simulink model "lab3_integration"  (R2020a)
settings: Solver=VariableStepAuto  StartTime=0.0  StopTime=10.0  RelTol=1e-3
libraries: androidsensorlib x3, sharedTrackingLibrary x1
settings Model: Creator=horia  LastModifiedBy=horia

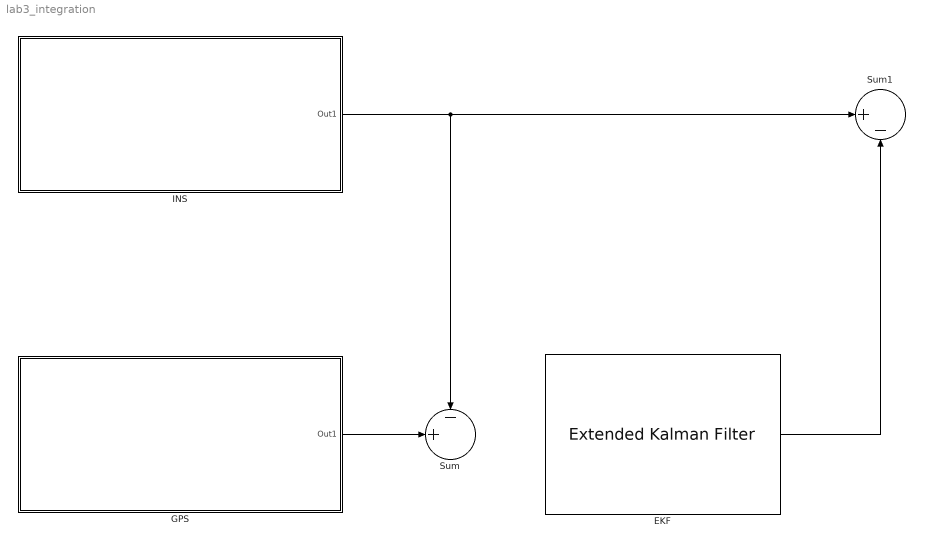
== system lab3_integration ==
  EKF : sharedTrackingLibrary/Extended Kalman Filter  StateTransitionFcn=myStateTransitionFcn  HasStateTransitionJacobianFcn=off  HasAdditiveProcessNoise=Additive  ProcessNoise=1  HasTimeVaryingProcessNoise=off  HasStateTransitionFcnExtraArgument=0  InitialState=0  InitialStateCovariance=1  MeasurementFcn1=myMeasurementFcn  HasMeasurementJacobianFcn1=off  HasMeasurementEnablePort1=off  HasAdditiveMeasurementNoise1=Additive  MeasurementNoise1=1  HasTimeVaryingMeasurementNoise1=off  HasMeasurementFcnExtraArgument1=0  MeasurementFcn2=myMeasurementFcn  HasMeasurementJacobianFcn2=off  HasMeasurementEnablePort2=off  HasAdditiveMeasurementNoise2=Additive  MeasurementNoise2=1  HasTimeVaryingMeasurementNoise2=off  HasMeasurementFcnExtraArgument2=0  MeasurementFcn3=myMeasurementFcn  HasMeasurementJacobianFcn3=off  HasMeasurementEnablePort3=off  HasAdditiveMeasurementNoise3=Additive  MeasurementNoise3=1  HasTimeVaryingMeasurementNoise3=off  HasMeasurementFcnExtraArgument3=0  MeasurementFcn4=myMeasurementFcn  HasMeasurementJacobianFcn4=off  HasMeasurementEnablePort4=off  HasAdditiveMeasurementNoise4=Additive  MeasurementNoise4=1  HasTimeVaryingMeasurementNoise4=off  HasMeasurementFcnExtraArgument4=0  MeasurementFcn5=myMeasurementFcn  HasMeasurementJacobianFcn5=off  HasMeasurementEnablePort5=off  HasAdditiveMeasurementNoise5=Additive  MeasurementNoise5=1  HasTimeVaryingMeasurementNoise5=off  HasMeasurementFcnExtraArgument5=0  EnableMultirate=off  StateTransitionFcnSampleTime=1  MeasurementFcn1SampleTime=1  MeasurementFcn2SampleTime=1  MeasurementFcn3SampleTime=1  MeasurementFcn4SampleTime=1  MeasurementFcn5SampleTime=1  UseCurrentEstimator=on  OutputStateCovariance=off  DataType=double  SampleTime=1  NumberOfMeasurements=2
      settings: SourceProductBaseCode=CT,DR,TF,ID,NV,AR,RO,VE
  GPS : Subsystem
  INS : Subsystem
  Sum : Sum  Inputs=-+|
  Sum1 : Sum  Inputs=|+-
  wires:
  GPS/1(Out1) -> Sum/2
  INS/1(Out1) -> Sum1/1, Sum/1
  EKF/1 -> Sum1/2

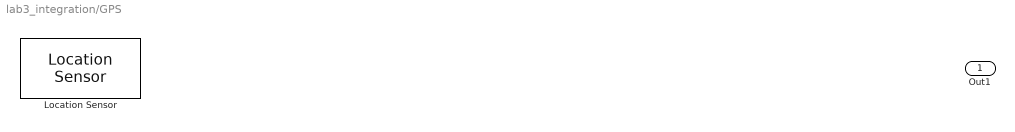
== system lab3_integration/GPS ==
  Location Sensor : androidsensorlib/Location Sensor  OutputVector=off  SampleTime=0.1  BlockPlatform=Android
      settings: SourceProductBaseCode=ANDROID
  Out1 : Outport

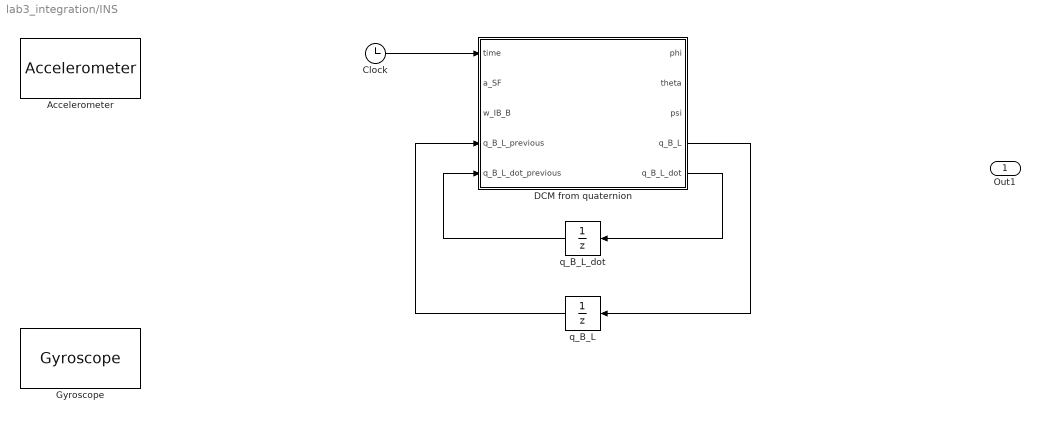
== system lab3_integration/INS ==
  Accelerometer : androidsensorlib/Accelerometer  OutputVector=off  SampleTime=0.1  BlockPlatform=Android
      settings: SourceProductBaseCode=ANDROID
  Clock : Clock
  DCM from quaternion : MATLAB Function  TreatAsAtomicUnit=on
  Gyroscope : androidsensorlib/Gyroscope  OutputVector=off  SampleTime=0.1  BlockPlatform=Android
      settings: SourceProductBaseCode=ANDROID
  q_B_L : UnitDelay  InitialCondition=[1;0;0;0]  SampleTime=-1  HasFrameUpgradeWarning=on
  q_B_L_dot : UnitDelay  InitialCondition=zeros(4,1)  SampleTime=-1  HasFrameUpgradeWarning=on
  Out1 : Outport
  wires:
  q_B_L_dot/1 -> DCM from quaternion/5(q_B_L_dot_previous)
  DCM from quaternion/4(q_B_L) -> q_B_L/1
  DCM from quaternion/5(q_B_L_dot) -> q_B_L_dot/1
  q_B_L/1 -> DCM from quaternion/4(q_B_L_previous)
  Clock/1 -> DCM from quaternion/1(time)

== matlab function lab3_integration/INS/DCM from quaternion ==
  data: time input; a_SF input; phi output; w_IB_B input; theta output; psi output; q_B_L_previous input; q_B_L_dot_previous input; q_B_L output; q_B_L_dot output
function [phi,theta,psi,q_B_L,q_B_L_dot] = fcn(time,a_SF,w_IB_B,q_B_L_previous,q_B_L_dot_previous)
%-- Partie initialisation ---------------------
persistent FlagInit counteur
theta = 0;
phi = 0;
psi = 0;
q_B_L = q_B_L_previous ;
q_B_L_dot = q_B_L_dot_previous  ;
a_SF_sum = zeros(1,3);

%%%%%%%%%%%%%%%%%%%%%%%%%%%%%%%%%%%%%%%%%%%%%%%%%%%%%%%%%%%%%%%%%%%%%%%%%%%
%
%  function R=q2dcm(q)
%
%>
%> @brief Function that converts a  quaternion vector to a directional
%> cosine matrix (rotation matrix) 
%>
%> @param[out]   R      Rotation matrix.
%> @param[in]    q      Quaternion vector.
%>
%
%%%%%%%%%%%%%%%%%%%%%%%%%%%%%%%%%%%%%%%%%%%%%%%%%%%%%%%%%%%%%%%%%%%%%%%%%%%
function R=q2dcm(q)

R = zeros(3,3);
p=zeros(6,1);

p(1:4)=q.^2;

p(5)=p(2)+p(3);

if p(1)+p(4)+p(5)~=0
   p(6)=2/(p(1)+p(4)+p(5)); 
else
   p(6)=0;
end


R(1,1)=1-p(6)*p(5);
R(2,2)=1-p(6)*(p(1)+p(3));
R(3,3)=1-p(6)*(p(1)+p(2));

p(1)=p(6)*q(1); 
p(2)=p(6)*q(2);
p(5)=p(6)*q(3)*q(4);
p(6)=p(1)*q(2);

R(1,2)=p(6)-p(5);
R(2,1)=p(6)+p(5);

p(5)=p(2)*q(4);
p(6)=p(1)*q(3);

R(1,3)=p(6)+p(5);
R(3,1)=p(6)-p(5);

p(5)=p(1)*q(4);
p(6)=p(2)*q(3);

R(2,3)=p(6)-p(5);
R(3,2)=p(6)+p(5);

end


%%%%%%%%%%%%%%%%%%%%%%%%%%%%%%%%%%%%%%%%%%%%%%%%%%%%%%%%%%%%%%%%%%%%%%%%%%%
%
%  function q=dcm2q(R)
%
%>
%> @brief Function that converts a directional cosine matrix (rotation 
%> matrix) in to a quaternion vector. 
%>
%> @param[out]    q      Quaternion vector.
%> @param[in]   R      Rotation matrix.
%>
%
%%%%%%%%%%%%%%%%%%%%%%%%%%%%%%%%%%%%%%%%%%%%%%%%%%%%%%%%%%%%%%%%%%%%%%%%%%%
function q=dcm2q(R)

T = 1 + R(1,1) + R(2,2) + R(3,3);

if T > 10^-8
    
    S = 0.5 / sqrt(T);
    qw = 0.25 / S;
    qx = ( R(3,2) - R(2,3) ) * S;
    qy = ( R(1,3) - R(3,1) ) * S;
    qz = ( R(2,1) - R(1,2) ) * S;

else
    
    if (R(1,1) > R(2,2)) && (R(1,1) > R(3,3))
        
        S = sqrt( 1 + R(1,1) - R(2,2) - R(3,3)) * 2; % S=4*qx
        qw = (R(3,2) - R(2,3)) / S;
        qx = 0.25 * S;
        qy = (R(1,2) + R(2,1)) / S;
        qz = (R(1,3) + R(3,1)) / S;
        
    elseif (R(2,2) > R(3,3))
        
        S = sqrt( 1 + R(2,2) - R(1,1) - R(3,3) ) * 2; %S=4*qy
        qw = (R(1,3) - R(3,1)) / S;
        qx = (R(1,2) + R(2,1)) / S;
        qy = 0.25 * S;
        qz = (R(2,3) + R(3,2)) / S;

    else
        
        S = sqrt( 1 + R(3,3) - R(1,1) - R(2,2) ) * 2; % S=4*qz
        qw = (R(2,1) - R(1,2)) / S;
        qx = (R(1,3) + R(3,1)) / S;
        qy = (R(2,3) + R(3,2)) / S;
        qz = 0.25 * S;

    end

end

%Store in vector
q = [qx qy qz qw]';
end



%-------------- La magnitude de l'acceleration est definie par :-----
accel_mag = sqrt(a_SF(1)^2 + a_SF(2)^2 + a_SF(3)^2);
%----------Par définition, l’axe Z du repère L est orienté selon gP
AxeZ_SF = - a_SF / accel_mag; 

%--------Init Matrix------------------
if isempty(FlagInit) && isempty(counteur)
%-- Initialisation des composentes Euler et la marice DCM
    a_SF_sum(1) =  AxeZ_SF(1);
    a_SF_sum(2) =  AxeZ_SF(2);
    a_SF_sum(3) =  AxeZ_SF(3);
%     for i = 1:3
%         a_SF_sum(i) = 0;
%     end
    FlagInit = 0;
    counteur = 0;
end

%En supposant que le système est stationnaire pendant les 25 premiers
%échantillons, le roulis et le tangage initiaux sont calculés à partir 
%des 25 premiers lectures de l'accéléromètre.
% Determination de l'Alttitude 
if (FlagInit == 0)
C_B_L = zeros(3);
%---- Initialisation par Alignement Grossier------
    C_B_L(3,1) = a_SF_sum(1);
    C_B_L(3,2) = a_SF_sum(2);
    C_B_L(3,3) = a_SF_sum(3);
    K = 1/sqrt(C_B_L(3,2)^2+C_B_L(3,3)^2);
    C_B_L(2,1) = 0;
    C_B_L(2,2) = K * C_B_L(3,3);
    C_B_L(2,3) =-K * C_B_L(3,2);
    C_B_L(1,1) = C_B_L(2,2) * C_B_L(3,3) - C_B_L(2,3) * C_B_L(3,2);
    C_B_L(1,2) = C_B_L(2,3) * C_B_L(3,1) - C_B_L(2,1) * C_B_L(3,3);
    C_B_L(1,3) = C_B_L(2,1) * C_B_L(3,2) - C_B_L(2,2) * C_B_L(3,1);
    C_B_L = [C_B_L(1,1) C_B_L(1,2) C_B_L(1,3); C_B_L(2,1) C_B_L(2,2) C_B_L(2,3); C_B_L(3,1) C_B_L(3,2) C_B_L(3,3)];
    %calculate initial quaternion from C_B_L matrix
    q_B_L = dcm2q(C_B_L);
    %calculate euler angles phi, theta, psi
    psi   = atan2( 2 *(q_B_L(2) * q_B_L(3) - q_B_L(1) * q_B_L(4)) , 2 * (q_B_L(1)^2 + q_B_L(1)^2) - 1 ) * 180/pi ;
    theta = -asin( 2 *(q_B_L(2) * q_B_L(4) + q_B_L(1) * q_B_L(3))) * 180/pi;
    phi   = atan2( 2* (q_B_L(3) * q_B_L(4) - q_B_L(1) * q_B_L(2)) , 2 * (q_B_L(1)^2 + q_B_L(4)^2) - 1 ) * 180/pi;
    FlagInit = 1;
elseif FlagInit == 1
%Create skew symetric matrix of gyroscope output
   Qw_B_IB_Mat =[    0       -w_IB_B(1)    -w_IB_B(2)    -w_IB_B(3);
                 w_IB_B(1)       0         -w_IB_B(3)     w_IB_B(2);
                 w_IB_B(2)    w_IB_B(3)         0        -w_IB_B(1);
                 w_IB_B(3)   -w_IB_B(2)     w_IB_B(1)          0    ];

    q_L_B = transpose([q_B_L(1) ;q_B_L(2); q_B_L(3); q_B_L(4)]);
%Variation du quaternion
    q_B_L_dot = 0.5 * Qw_B_IB_Mat * q_B_L;
    q_B_L_dot = [ q_B_L_dot(1); q_B_L_dot(2); q_B_L_dot(3); q_B_L_dot(4)];
%trapezoidal integration to get new q_B_L 
%---- Équations de propagation d'attitude             
%---- Trapezoide integre q_B_L
    q_B_L = q_B_L_previous + (0.01/2) *( q_B_L_dot + q_B_L_dot_previous );
    C_B_N = q2dcm(q_B_L);
%Calcule de la variation d'Attitude Quaternion 
    psi   = atan2( 2 *(q_B_L(2) * q_B_L(3) - q_B_L(1) * q_B_L(4)) , 2 * (q_B_L(1)^2 + q_B_L(2)^2) - 1 ) * 180/pi ;
    theta = -asin( 2 *(q_B_L(2) * q_B_L(4) + q_B_L(1) * q_B_L(3))) * 180/pi;
    phi   = atan2( 2* (q_B_L(3) * q_B_L(4) - q_B_L(1) * q_B_L(2)) , 2 * (q_B_L(1)^2 + q_B_L(4)^2) - 1 ) * 180/pi;
%Calcule de l'acceleration 
    
    
    
end

end
